simulink model "BrowarModel"  (R2024a)
settings: Solver=ode5  StartTime=0.0  StopTime=inf  FixedStep=0.1  RelTol=1e-3
undefined symbols (not defined in the file or in its folder): localhost, Matrikon, OI
libraries: opclib x24
(part 6 of 9)

== system BrowarModel/Mlyn browarniany/Mlyn browarniany/Zawor doplywu slodu ==
  note: Zawor doplywu slodu
  note: Uszkodzenie:
      | Brak materialu
  note: Uszkodzenie:
      | Dlawienie przeplywu w zaworze
  note: Uszkodzenie:
      | Przeciek wewnetrzny w zaworze
  note: Uszkodzenie:
      | Wyciek zewnetrzny w zaworze
  Sterowanie : Inport
  Dlawienie : Inport  Port=2
  Przeciek : Inport  Port=3
  Wyciek : Inport  Port=4
  Brak : Inport  Port=5
  Const : Constant  Value=100
  Const1 : Constant  Value=100
  Const2 : Constant  Value=100
  GUIMon : Gain
  Gain : Gain  Gain=1/100
  Gain1 : Gain  Gain=1/100
  Gain2 : Gain  Gain=1/100
  Integer Delay : Delay  DelayLength=15
  Napelnianie m3/s : Gain  Gain=Fmax/100
  Product : Product  RndMeth=Zero
  Product1 : Product  RndMeth=Zero
  Product2 : Product  RndMeth=Zero
  Relay : Relay  OnOutputValue=100
  Sat (0-100) : Saturate  UpperLimit=100  LowerLimit=0
  Sat dlawienie (0-100) : Saturate  UpperLimit=100  LowerLimit=0
  Sat przecieku (0-100) : Saturate  UpperLimit=100  LowerLimit=0
  Sat uszk (0-100) : Saturate  UpperLimit=100  LowerLimit=0
  Sat wyciek (0-100) : Saturate  UpperLimit=100  LowerLimit=0
  Sum : Sum  Inputs=|+-
  Sum1 : Sum  Inputs=|++
  Sum2 : Sum  Inputs=|+-
  Sum3 : Sum  Inputs=|+-
  Sum5 : Sum  Inputs=|++
  Transfer Fcn : TransferFcn  Denominator=[1 1]
  Zaklocenia : Subsystem
  Przeplyw : Outport
  wires:
  Product/1 -> Transfer Fcn/1  "m3/s"
  Const/1 -> Sum/1
  Sat dlawienie (0-100)/1 -> Sum/2
  Sum/1 -> Gain/1
  Transfer Fcn/1 -> Integer Delay/1  "m3/s"
  Sterowanie/1 -> Relay/1
  Dlawienie/1 -> Sat dlawienie (0-100)/1  "[0,100]"
  Sat (0-100)/1 -> Napelnianie m3/s/1
  Sum1/1 -> Sat (0-100)/1
  Relay/1 -> GUIMon/1
  Przeciek/1 -> Sat przecieku (0-100)/1
  Sat przecieku (0-100)/1 -> Sum1/2
  Wyciek/1 -> Sat wyciek (0-100)/1
  Const1/1 -> Sum2/1
  Sat wyciek (0-100)/1 -> Sum2/2
  Integer Delay/1 -> Product1/1  "m3/s"
  Product1/1 -> Przeplyw/1
  Sum2/1 -> Gain1/1
  Gain1/1 -> Product1/2
  Product2/1 -> Sum1/1
  GUIMon/1 -> Product2/2
  Brak/1 -> Sat uszk (0-100)/1
  Const2/1 -> Sum3/1
  Sat uszk (0-100)/1 -> Sum3/2
  Sum3/1 -> Gain2/1
  Sum5/1 -> Product/2
  Gain/1 -> Product/1
  Zaklocenia/1(Out) -> Sum5/2
  Gain2/1 -> Product2/1
  Napelnianie m3/s/1 -> Sum5/1, Zaklocenia/1(In)

== system BrowarModel/Mlyn browarniany/ST103/Zaklocenia pomiarowe ==
  Product1 : Product  InputSameDT=on  RndMeth=Zero  SaturateOnIntegerOverflow=on  OutDataTypeStr=Inherit: Same as first input
  Product3 : Product  InputSameDT=on  RndMeth=Zero  SaturateOnIntegerOverflow=on  OutDataTypeStr=Inherit: Same as first input
  Random Number : RandomNumber  Variance=.5  Seed=4365624  SampleTime=0.1
  Transfer Fcn1 : TransferFcn  Denominator=[0.5 1]
  Transfer Fcn2 : TransferFcn  Denominator=[0.5 1]
  Zaklocenia pomiarowe : Constant  Value=ZakloceniaPom
  Out : Outport
  wires:
  Random Number/1 -> Product3/1
  Product3/1 -> Transfer Fcn1/1
  Transfer Fcn1/1 -> Transfer Fcn2/1
  Transfer Fcn2/1 -> Out/1
  Zaklocenia pomiarowe/1 -> Product1/2
  [ZaklPom] -> Product1/1
  Product1/1 -> Product3/2

== system BrowarModel/Mlyn browarniany/ST105/Zaklocenia pomiarowe ==
  Product1 : Product  InputSameDT=on  RndMeth=Zero  SaturateOnIntegerOverflow=on  OutDataTypeStr=Inherit: Same as first input
  Product3 : Product  InputSameDT=on  RndMeth=Zero  SaturateOnIntegerOverflow=on  OutDataTypeStr=Inherit: Same as first input
  Random Number : RandomNumber  Variance=.5  Seed=4365624  SampleTime=0.1
  Transfer Fcn1 : TransferFcn  Denominator=[0.5 1]
  Transfer Fcn2 : TransferFcn  Denominator=[0.5 1]
  Zaklocenia pomiarowe : Constant  Value=ZakloceniaPom
  Out : Outport
  wires:
  Product1/1 -> Product3/2
  [ZaklPom] -> Product1/1
  Zaklocenia pomiarowe/1 -> Product1/2
  Transfer Fcn2/1 -> Out/1
  Transfer Fcn1/1 -> Transfer Fcn2/1
  Product3/1 -> Transfer Fcn1/1
  Random Number/1 -> Product3/1

== system BrowarModel/Mlyn browarniany/TT103/Zaklocenia pomiarowe ==
  Product1 : Product  InputSameDT=on  RndMeth=Zero  SaturateOnIntegerOverflow=on  OutDataTypeStr=Inherit: Same as first input
  Product3 : Product  InputSameDT=on  RndMeth=Zero  SaturateOnIntegerOverflow=on  OutDataTypeStr=Inherit: Same as first input
  Random Number : RandomNumber  Variance=.5  Seed=4365624  SampleTime=0.1
  Transfer Fcn1 : TransferFcn  Denominator=[0.5 1]
  Transfer Fcn2 : TransferFcn  Denominator=[0.5 1]
  Zaklocenia pomiarowe : Constant  Value=ZakloceniaPom
  Out : Outport
  wires:
  Random Number/1 -> Product3/1
  Product3/1 -> Transfer Fcn1/1
  Transfer Fcn1/1 -> Transfer Fcn2/1
  Transfer Fcn2/1 -> Out/1
  Zaklocenia pomiarowe/1 -> Product1/2
  [ZaklPom] -> Product1/1
  Product1/1 -> Product3/2

== system BrowarModel/Mlyn browarniany/TT105/Zaklocenia pomiarowe ==
  Product1 : Product  InputSameDT=on  RndMeth=Zero  SaturateOnIntegerOverflow=on  OutDataTypeStr=Inherit: Same as first input
  Product3 : Product  InputSameDT=on  RndMeth=Zero  SaturateOnIntegerOverflow=on  OutDataTypeStr=Inherit: Same as first input
  Random Number : RandomNumber  Variance=.5  Seed=4365624  SampleTime=0.1
  Transfer Fcn1 : TransferFcn  Denominator=[0.5 1]
  Transfer Fcn2 : TransferFcn  Denominator=[0.5 1]
  Zaklocenia pomiarowe : Constant  Value=ZakloceniaPom
  Out : Outport
  wires:
  Product1/1 -> Product3/2
  [ZaklPom] -> Product1/1
  Zaklocenia pomiarowe/1 -> Product1/2
  Transfer Fcn2/1 -> Out/1
  Transfer Fcn1/1 -> Transfer Fcn2/1
  Product3/1 -> Transfer Fcn1/1
  Random Number/1 -> Product3/1

== system BrowarModel/Schladzacz/TT601/Zaklocenia pomiarowe ==
  Product1 : Product  InputSameDT=on  RndMeth=Zero  SaturateOnIntegerOverflow=on  OutDataTypeStr=Inherit: Same as first input
  Product3 : Product  InputSameDT=on  RndMeth=Zero  SaturateOnIntegerOverflow=on  OutDataTypeStr=Inherit: Same as first input
  Random Number : RandomNumber  Variance=.5  Seed=4365624  SampleTime=0.1
  Transfer Fcn1 : TransferFcn  Denominator=[0.5 1]
  Transfer Fcn2 : TransferFcn  Denominator=[0.5 1]
  Zaklocenia pomiarowe : Constant  Value=ZakloceniaPom
  Out : Outport
  wires:
  Random Number/1 -> Product3/1
  Product3/1 -> Transfer Fcn1/1
  Transfer Fcn1/1 -> Transfer Fcn2/1
  Transfer Fcn2/1 -> Out/1
  Zaklocenia pomiarowe/1 -> Product1/2
  [ZaklPom] -> Product1/1
  Product1/1 -> Product3/2

== system BrowarModel/Schladzacz/TT602/Zaklocenia pomiarowe ==
  Product1 : Product  InputSameDT=on  RndMeth=Zero  SaturateOnIntegerOverflow=on  OutDataTypeStr=Inherit: Same as first input
  Product3 : Product  InputSameDT=on  RndMeth=Zero  SaturateOnIntegerOverflow=on  OutDataTypeStr=Inherit: Same as first input
  Random Number : RandomNumber  Variance=.5  Seed=4365624  SampleTime=0.1
  Transfer Fcn1 : TransferFcn  Denominator=[0.5 1]
  Transfer Fcn2 : TransferFcn  Denominator=[0.5 1]
  Zaklocenia pomiarowe : Constant  Value=ZakloceniaPom
  Out : Outport
  wires:
  Product1/1 -> Product3/2
  [ZaklPom] -> Product1/1
  Zaklocenia pomiarowe/1 -> Product1/2
  Transfer Fcn2/1 -> Out/1
  Transfer Fcn1/1 -> Transfer Fcn2/1
  Product3/1 -> Transfer Fcn1/1
  Random Number/1 -> Product3/1

== system BrowarModel/Schladzacz/TT603/Zaklocenia pomiarowe ==
  Product1 : Product  InputSameDT=on  RndMeth=Zero  SaturateOnIntegerOverflow=on  OutDataTypeStr=Inherit: Same as first input
  Product3 : Product  InputSameDT=on  RndMeth=Zero  SaturateOnIntegerOverflow=on  OutDataTypeStr=Inherit: Same as first input
  Random Number : RandomNumber  Variance=.5  Seed=4365624  SampleTime=0.1
  Transfer Fcn1 : TransferFcn  Denominator=[0.5 1]
  Transfer Fcn2 : TransferFcn  Denominator=[0.5 1]
  Zaklocenia pomiarowe : Constant  Value=ZakloceniaPom
  Out : Outport
  wires:
  Random Number/1 -> Product3/1
  Product3/1 -> Transfer Fcn1/1
  Transfer Fcn1/1 -> Transfer Fcn2/1
  Transfer Fcn2/1 -> Out/1
  Zaklocenia pomiarowe/1 -> Product1/2
  [ZaklPom] -> Product1/1
  Product1/1 -> Product3/2

== system BrowarModel/Schladzacz/TT604/Zaklocenia pomiarowe ==
  Product1 : Product  InputSameDT=on  RndMeth=Zero  SaturateOnIntegerOverflow=on  OutDataTypeStr=Inherit: Same as first input
  Product3 : Product  InputSameDT=on  RndMeth=Zero  SaturateOnIntegerOverflow=on  OutDataTypeStr=Inherit: Same as first input
  Random Number : RandomNumber  Variance=.5  Seed=4365624  SampleTime=0.1
  Transfer Fcn1 : TransferFcn  Denominator=[0.5 1]
  Transfer Fcn2 : TransferFcn  Denominator=[0.5 1]
  Zaklocenia pomiarowe : Constant  Value=ZakloceniaPom
  Out : Outport
  wires:
  Product1/1 -> Product3/2
  [ZaklPom] -> Product1/1
  Zaklocenia pomiarowe/1 -> Product1/2
  Transfer Fcn2/1 -> Out/1
  Transfer Fcn1/1 -> Transfer Fcn2/1
  Product3/1 -> Transfer Fcn1/1
  Random Number/1 -> Product3/1

== system BrowarModel/System dozowania chmielu/PT503/Zaklocenia pomiarowe ==
  Product1 : Product  InputSameDT=on  RndMeth=Zero  SaturateOnIntegerOverflow=on  OutDataTypeStr=Inherit: Same as first input
  Product3 : Product  InputSameDT=on  RndMeth=Zero  SaturateOnIntegerOverflow=on  OutDataTypeStr=Inherit: Same as first input
  Random Number : RandomNumber  Variance=.5  Seed=4365624  SampleTime=0.1
  Transfer Fcn1 : TransferFcn  Denominator=[0.5 1]
  Transfer Fcn2 : TransferFcn  Denominator=[0.5 1]
  Zaklocenia pomiarowe : Constant  Value=ZakloceniaPom
  Out : Outport
  wires:
  Product1/1 -> Product3/2
  [ZaklPom] -> Product1/1
  Zaklocenia pomiarowe/1 -> Product1/2
  Transfer Fcn2/1 -> Out/1
  Transfer Fcn1/1 -> Transfer Fcn2/1
  Product3/1 -> Transfer Fcn1/1
  Random Number/1 -> Product3/1

== system BrowarModel/System dozowania chmielu/System dozowania chmielu/Ruszt dozujacy ==
  note: Ruszt dozujacy
  Pozycja : Inport
  Poziom_w_zbiorniku : Inport  Port=2
  Dot Product : DotProduct  OutDataTypeStr=Inherit: Inherit via internal rule
  Gain : Gain  Gain=20
  Inercja proszku : TransferFcn  Denominator=[0.1 1]
  Parcie proszku na ruszt : Lookup  InputValues=[0, 0.1, 5]  Table=[0, 1, 1]  SaturateOnIntegerOverflow=off
  Pole otwarcia : Lookup  InputValues=[0, 0.015, 0.05, 0.09, 0.1]  Table=[0, 0, 0.0003, 0.001, 0.001]  SaturateOnIntegerOverflow=off
  Saturation : Saturate  UpperLimit=inf  LowerLimit=0
  Przeplyw : Outport
  wires:
  Pozycja/1 -> Pole otwarcia/1  "m"
  Pole otwarcia/1 -> Gain/1
  Poziom_w_zbiorniku/1 -> Parcie proszku na ruszt/1  "m"
  Parcie proszku na ruszt/1 -> Dot Product/2
  Dot Product/1 -> Inercja proszku/1  "m^3/s"
  Inercja proszku/1 -> Saturation/1  "m3/s"
  Saturation/1 -> Przeplyw/1
  Gain/1 -> Dot Product/1

== system BrowarModel/System dozowania chmielu/System dozowania chmielu/Silownik hydrauliczny ==
  note: Silownik hydrauliczny
  Przeplyw zasilanie : Inport
  Uszkodzenie : Inport  Port=2
  Abs1 : Abs  SaturateOnIntegerOverflow=off
  Abs2 : Abs  SaturateOnIntegerOverflow=off
  Add : Sum
  Add1 : Sum
  Add2 : Sum
  Brak przeplywu : Constant  Value=0
  Divide1 : Product  Inputs=*/
  Divide2 : Product  Inputs=/*
  Dot Product : DotProduct  OutDataTypeStr=Inherit: Inherit via internal rule
  Dot Product1 : DotProduct  OutDataTypeStr=Inherit: Inherit via internal rule
  Gain : Gain  Gain=0.1/100
  Inercja : TransferFcn  Denominator=[0.2 1]
  Integrator : Integrator  LimitOutput=on  UpperSaturationLimit=0.1  LowerSaturationLimit=0  ShowSaturationPort=on
  Napelnianie : Saturate  UpperLimit=inf  LowerLimit=0
  Napelnianie1 : Saturate  UpperLimit=inf  LowerLimit=0
  Oproznianie : Saturate  UpperLimit=0  LowerLimit=-inf
  Oproznianie1 : Saturate  UpperLimit=0  LowerLimit=-inf
  Pole tloczyska gdy silownik otwierany : Constant  Value=0.002
  Pole tloczyska gdy silownik zamykany : Constant  Value=0.001
  Sat : Saturate  UpperLimit=100  LowerLimit=0
  Sat1 : Saturate  UpperLimit=0.1  LowerLimit=0
  Switch : Switch  Threshold=0.5  SaturateOnIntegerOverflow=off  InputSameDT=off
  Pozycja : Outport
  Przeplyw pobor : Outport  Port=2
  wires:
  Przeplyw zasilanie/1 -> Napelnianie/1, Oproznianie/1  "m3/s"
  Add/1 -> Inercja/1  "m/s"
  Napelnianie/1 -> Divide2/2
  Divide2/1 -> Add/1  "m/s"
  Divide1/1 -> Add/2  "m/s"
  Oproznianie/1 -> Divide1/1
  Pole tloczyska gdy silownik zamykany/1 -> Divide1/2, Dot Product1/2
  Pole tloczyska gdy silownik otwierany/1 -> Divide2/1, Dot Product/1
  Switch/1 -> Przeplyw pobor/1
  Integrator/2 -> Abs2/1
  Inercja/1 -> Integrator/1, Napelnianie1/1, Oproznianie1/1
  Oproznianie1/1 -> Abs1/1
  Abs1/1 -> Dot Product1/1
  Napelnianie1/1 -> Dot Product/2
  Dot Product/1 -> Add1/1
  Abs2/1 -> Switch/2
  Brak przeplywu/1 -> Switch/1
  Add1/1 -> Switch/3
  Dot Product1/1 -> Add1/2
  Uszkodzenie/1 -> Sat/1
  Integrator/1 -> Add2/2  "m"
  Add2/1 -> Sat1/1
  Sat/1 -> Gain/1
  Sat1/1 -> Pozycja/1
  Gain/1 -> Add2/1

== system BrowarModel/System dozowania chmielu/System dozowania chmielu/Sterownik rusztu ==
  note: Sterownik rusztu
  Pozycja rusztu : Inport
  Nastawa : Inport  Port=2
  Char rusztu (reset) : Lookup  InputValues=|  Table=|  SaturateOnIntegerOverflow=off
      InputValues=|
      | [1
      | 2
      | 3
      | 4
      | 5
      | 6
      | 7
      | 8
      | 9
      | 10
      | 11
      | 12
      | 13
      | 14
      | 15
      | 16
      | 17
      | 18
      | 19
      | 20
      | 21
      | 22
      | 23
      | 24
      | 25
      | 26
      | 27
      | 28
      | 29
      | 30
      | 31
      | 32
      | 33
      | 34
      | 35
      | 36
      | 37
      | 38
      | 39
      | 40
      | 41
      | 42
      | 43
      | 44
      | 45
      | 46
      | 47
      | 48
      | 49
      | 50
      | 51
      | 52
      | 53
      | 54
      | 55
      | 56
      | 57
      | 58
      | 59
      | 60
      | 61
      | 62
      | 63
      | 64
      | 65
      | 66
      | 67
      | 68
      | 69
      | 70
      | 71
      | 72
      | 73
      | 74
      | 75
      | 76
      | 77
      | 78
      | 79
      | 80
      | 81
      | 82
      | 83
      | 84
      | 85
      | 86
      | 87
      | 88
      | 89
      | 90
      | 91
      | 92
      | 93
      | 94
      | 95
      | 96
      | 97
      | 98
      | 99
      | 100]
      Table=|
      | [9.24
      | 9.55
      | 9.84
      | 10.13
      | 10.44
      | 10.76
      | 11.11
      | 11.47
      | 11.84
      | 12.24
      | 12.65
      | 13.08
      | 13.52
      | 13.98
      | 14.45
      | 14.94
      | 15.44
      | 15.95
      | 16.48
      | 17.02
      | 17.58
      | 18.15
      | 18.72
      | 19.32
      | 19.92
      | 20.53
      | 21.16
      | 21.80
      | 22.44
      | 23.10
      | 23.77
      | 24.45
      | 25.14
      | 25.84
      | 26.56
      | 27.28
      | 28.01
      | 28.75
      | 29.50
      | 30.26
      | 31.03
      | 31.80
      | 32.59
      | 33.39
      | 34.19
      | 35.00
      | 35.83
      | 36.66
      | 37.50
      | 38.35
      | 39.20
      | 40.07
      | 40.94
      | 41.82
      | 42.71
      | 43.61
      | 44.51
      | 45.42
      | 46.35
      | 47.27
      | 48.21
      | 49.15
      | 50.10
      | 51.06
      | 52.03
      | 53.00
      | 53.98
      | 54.97
      | 55.97
      | 56.97
      | 57.98
      | 59.00
      | 60.02
      | 61.05
      | 62.09
      | 63.13
      | 64.18
      | 65.24
      | 66.31
      | 67.38
      | 68.46
      | 69.54
      | 70.63
      | 71.73
      | 72.84
      | 73.95
      | 75.06
      | 76.19
      | 77.32
      | 78.46
      | 79.60
      | 80.75
      | 81.90
      | 83.06
      | 84.23
      | 85.40
      | 86.58
      | 87.77
      | 88.96
      | 90.16]
  Char rusztu (set) : Lookup  InputValues=|  Table=|  SaturateOnIntegerOverflow=off
      InputValues=|
      | [1
      | 2
      | 3
      | 4
      | 5
      | 6
      | 7
      | 8
      | 9
      | 10
      | 11
      | 12
      | 13
      | 14
      | 15
      | 16
      | 17
      | 18
      | 19
      | 20
      | 21
      | 22
      | 23
      | 24
      | 25
      | 26
      | 27
      | 28
      | 29
      | 30
      | 31
      | 32
      | 33
      | 34
      | 35
      | 36
      | 37
      | 38
      | 39
      | 40
      | 41
      | 42
      | 43
      | 44
      | 45
      | 46
      | 47
      | 48
      | 49
      | 50
      | 51
      | 52
      | 53
      | 54
      | 55
      | 56
      | 57
      | 58
      | 59
      | 60
      | 61
      | 62
      | 63
      | 64
      | 65
      | 66
      | 67
      | 68
      | 69
      | 70
      | 71
      | 72
      | 73
      | 74
      | 75
      | 76
      | 77
      | 78
      | 79
      | 80
      | 81
      | 82
      | 83
      | 84
      | 85
      | 86
      | 87
      | 88
      | 89
      | 90
      | 91
      | 92
      | 93
      | 94
      | 95
      | 96
      | 97
      | 98
      | 99
      | 100]
      Table=|
      | [7.50
      | 7.66
      | 7.80
      | 7.95
      | 8.10
      | 8.26
      | 8.43
      | 8.61
      | 8.80
      | 9.00
      | 9.20
      | 9.42
      | 9.64
      | 9.87
      | 10.11
      | 10.35
      | 10.60
      | 10.86
      | 11.12
      | 11.39
      | 11.67
      | 11.95
      | 12.24
      | 12.54
      | 12.84
      | 13.15
      | 13.46
      | 13.78
      | 14.10
      | 14.43
      | 14.77
      | 15.11
      | 15.45
      | 15.80
      | 16.16
      | 16.52
      | 16.88
      | 17.25
      | 17.63
      | 18.01
      | 18.39
      | 18.78
      | 19.17
      | 19.57
      | 19.98
      | 20.38
      | 20.79
      | 21.21
      | 21.63
      | 22.05
      | 22.48
      | 22.91
      | 23.35
      | 23.79
      | 24.23
      | 24.68
      | 25.14
      | 25.59
      | 26.05
      | 26.52
      | 26.98
      | 27.46
      | 27.93
      | 28.41
      | 28.89
      | 29.38
      | 29.87
      | 30.37
      | 30.86
      | 31.37
      | 31.87
      | 32.38
      | 32.89
      | 33.41
      | 33.92
      | 34.45
      | 34.97
      | 35.50
      | 36.03
      | 36.57
      | 37.11
      | 37.65
      | 38.20
      | 38.75
      | 39.30
      | 39.85
      | 40.41
      | 40.97
      | 41.54
      | 42.11
      | 42.68
      | 43.25
      | 43.83
      | 44.41
      | 45.00
      | 45.58
      | 46.17
      | 46.77
      | 47.36
      | 47.96]
  Constant : Constant  Value=0
  Gain : Gain  Gain=0.001
  Gain1 : Gain  Gain=0.001
  Logical Operator : Logic  Operator=OR  AllPortsSameDT=off
  Logical Operator1 : Logic  AllPortsSameDT=off
  Logical Operator2 : Logic  Operator=NOT  AllPortsSameDT=off
  Logical Operator3 : Logic  AllPortsSameDT=off
  Memory : Memory
  Relational Operator : RelationalOperator  Operator=<=  InputSameDT=off
  Relational Operator1 : RelationalOperator  InputSameDT=off
  Relational Operator2 : RelationalOperator  Operator=>  InputSameDT=off
  Rounding Function : Rounding
  Sterowanie zaworem : Outport
  wires:
  Nastawa/1 -> Rounding Function/1
  Char rusztu (set)/1 -> Gain/1  "%"
  Char rusztu (reset)/1 -> Gain1/1  "%"
  Relational Operator/1 -> Logical Operator/1
  Logical Operator/1 -> Memory/1, Logical Operator3/1
  Memory/1 -> Logical Operator1/1
  Logical Operator1/1 -> Logical Operator/2
  Relational Operator1/1 -> Logical Operator2/1
  Logical Operator2/1 -> Logical Operator1/2
  Pozycja rusztu/1 -> Relational Operator/1, Relational Operator1/1  "m"
  Logical Operator3/1 -> Sterowanie zaworem/1
  Relational Operator2/1 -> Logical Operator3/2
  Constant/1 -> Relational Operator2/2
  Gain/1 -> Relational Operator/2  "m"
  Gain1/1 -> Relational Operator1/2  "m"
  Rounding Function/1 -> Char rusztu (set)/1, Char rusztu (reset)/1, Relational Operator2/1

== system BrowarModel/System dozowania chmielu/System dozowania chmielu/Waga ==
  note: Waga
  note: Uszkodzenie mechanizmu
      | oprozniania wago
  Doplyw : Inport
  Oproznianie : Inport  Port=2
  Uszkodzenie oprozniania : Inport  Port=3
  1/Gestosc : Gain  Gain=1/1000
  Dot Product : DotProduct  OutDataTypeStr=Inherit: Inherit via internal rule
  Dynamika oprozniania : Gain  Gain=0.75
  Gestosc : Gain  Gain=1000
  Integrator : Integrator  LimitOutput=on  UpperSaturationLimit=100  LowerSaturationLimit=0
  Logical Operator : Logic  Operator=NOT  AllPortsSameDT=off
  Poz_dol : RelationalOperator  InputSameDT=off
  Poz_gora : RelationalOperator  Operator=<=  InputSameDT=off
  Pozycja dol : Constant  Value=0.9
  Pozycja gora : Constant  Value=0.1
  Product : Product  RndMeth=Zero
  Relay : Relay
  Relay1 : Relay
  Saturation : Saturate  UpperLimit=inf  LowerLimit=0
  Saturation1 : Saturate  UpperLimit=100  LowerLimit=0
  Sum : Sum  Inputs=|+-
  Sum1 : Sum
  Transfer Fcn : TransferFcn  Denominator=[1 1]
  Transport Delay : TransportDelay  DelayTime=1.5
  Wspolczynnik dynamiczny : Gain  Gain=.2
  Masa : Outport
  Odplyw chmielu : Outport  Port=2
  Poz dol : Outport  Port=3
  Poz gora : Outport  Port=4
  wires:
  Gestosc/1 -> Transport Delay/1  "kg/s"
  Transport Delay/1 -> Wspolczynnik dynamiczny/1, Sum/1
  Saturation/1 -> Gestosc/1  "m^3/s"
  Integrator/1 -> Dynamika oprozniania/1, Sum1/2
  Wspolczynnik dynamiczny/1 -> Sum1/1
  Doplyw/1 -> Saturation/1
  Sum1/1 -> Saturation1/1  "kg"
  Sum/1 -> Integrator/1
  Dot Product/1 -> Sum/2, 1/Gestosc/1
  Dynamika oprozniania/1 -> Dot Product/2
  1/Gestosc/1 -> Odplyw chmielu/1
  Saturation1/1 -> Masa/1  "kg"
  Poz_dol/1 -> Poz dol/1, Dot Product/1
  Poz_gora/1 -> Poz gora/1
  Pozycja dol/1 -> Poz_dol/2
  Pozycja gora/1 -> Poz_gora/2
  Transfer Fcn/1 -> Poz_dol/1, Poz_gora/1
  Oproznianie/1 -> Relay/1
  Uszkodzenie oprozniania/1 -> Relay1/1
  Relay1/1 -> Logical Operator/1
  Product/1 -> Transfer Fcn/1
  Relay/1 -> Product/1
  Logical Operator/1 -> Product/2

== system BrowarModel/System dozowania chmielu/System dozowania chmielu/Zasilacz hydrauliczny ==
  note: obr/min
  note: Zasilacz hydrauliczny
  note: Uszkodzenie:
      | Spadek cisnienia zasilania
  note: Uszkodzenie silnika pompy
  Zalaczenie pompy : Inport
  Przeplyw_pobor : Inport  Port=2
  Spadek cisnienia : Inport  Port=3
  Uszkodzenie silnika : Inport  Port=4
  Charakterystyka pompy F=f(P) (max 0.0001 m^3/s) : Lookup  InputValues=[0, 300]  Table=[0,0.0001]  SaturateOnIntegerOverflow=off
  Charakterystyka pompy P=f(obr) (max 300 kPa) : Lookup  InputValues=[0, 1440]  Table=[0,300]  SaturateOnIntegerOverflow=off
  Const1 : Constant  Value=100
  GUIMon : Gain
  Gain : Gain  Gain=1/100
  Gain1 : Gain  Gain=1/100
  Inercja wirnika : TransferFcn  Denominator=[0.5 1]
  Math Function : Math  Operator=square  SignedPower=on
  Obroty nominalne pompy : Gain  Gain=1440
  Opor : Gain  Gain=250 / ((0.0001)^2)
  Product1 : Product  RndMeth=Zero
  Relay : Relay  OnOutputValue=100
  Relay1 : Relay  OnOutputValue=0  OffOutputValue=1
  Sat uszk : Saturate  UpperLimit=100  LowerLimit=0
  Saturation : Saturate  UpperLimit=inf  LowerLimit=0
  Spadek obrotow pompy (od obciazenia) : Lookup  InputValues=[0, 300]  Table=[0,100]  SaturateOnIntegerOverflow=off
  Sum1 : Sum  Inputs=|+-
  Sum2 : Sum  Inputs=|+-
  Sum3 : Sum  Inputs=|+-
  Wplyw uszkodzenia : DotProduct  OutDataTypeStr=Inherit: Inherit via internal rule
  Max przeplyw zasilanie : Outport
  Cisnienie zasilania : Outport  Port=2
  wires:
  Obroty nominalne pompy/1 -> Sum2/1
  Sum2/1 -> Inercja wirnika/1
  Spadek obrotow pompy (od obciazenia)/1 -> Sum2/2  "obr/min"
  Inercja wirnika/1 -> Charakterystyka pompy P=f(obr) (max 300 kPa)/1  "obr/min"
  Charakterystyka pompy F=f(P) (max 0.0001 m^3/s)/1 -> Max przeplyw zasilanie/1  "m^3/s"
  Sum1/1 -> Saturation/1
  Opor/1 -> Sum1/2  "kPa"
  Saturation/1 -> Spadek obrotow pompy (od obciazenia)/1, Cisnienie zasilania/1, Charakterystyka pompy F=f(P) (max 0.0001 m^3/s)/1  "kPa"
  Math Function/1 -> Opor/1
  Zalaczenie pompy/1 -> Relay/1
  Przeplyw_pobor/1 -> Math Function/1
  Spadek cisnienia/1 -> Sat uszk/1
  Charakterystyka pompy P=f(obr) (max 300 kPa)/1 -> Product1/2  "kPa"
  Product1/1 -> Sum1/1  "kPa"
  Sat uszk/1 -> Sum3/2
  Const1/1 -> Sum3/1
  Sum3/1 -> Gain/1
  Wplyw uszkodzenia/1 -> Obroty nominalne pompy/1
  Relay/1 -> GUIMon/1
  Uszkodzenie silnika/1 -> Relay1/1
  Relay1/1 -> Wplyw uszkodzenia/2
  Gain/1 -> Product1/1
  GUIMon/1 -> Gain1/1
  Gain1/1 -> Wplyw uszkodzenia/1

== system BrowarModel/System dozowania chmielu/System dozowania chmielu/Zasobnik ==
  note: Zasobnik dozownika chmielu
  note: Uszkodzenie:
      | Wyciek z zasobnika dozownika
  Doplyw : Inport
  Odplyw : Inport  Port=2
  Wyciek : Inport  Port=3
  Char. zbiornika : Lookup  InputValues="[0.000\t0.003\t0.010\t0.023\t0.046\t0.079\t0.125\t0.186\t0.264\t0.362\t0.480\t0.622\t0.790\t0.972\t1.172\t1.372\t1.572\t1.772\t1.972\t2.172\t2.372\t2.572\t2.772\t2.972\t3.172\t3.372\t3.572\t3.772\t3.972\t4.172\t4.372\t4.572\t4.772\t4.972]"  Table="[0\t0.1\t0.2\t0.3\t0.4\t0.5\t0.6\t0.7\t0.8\t0.9\t1\t1.1\t1.2\t1.3\t1.4\t1.5\t1.6\t1.7\t1.8\t1.9\t2\t2.1\t2.2\t2.3\t2.4\t2.5\t2.6\t2.7\t2.8\t2.9\t3\t3.1\t3.2\t3.3]"  SaturateOnIntegerOverflow=off
  Detektory poziomu : Subsystem
  Integrator (max = 4.92m3) : Integrator  LimitOutput=on  UpperSaturationLimit=4.92  LowerSaturationLimit=0
  Max wyciek : Gain  Gain=0.01
  Product : Product  RndMeth=Zero
  Sat doplyw (F>=0) : Saturate  UpperLimit=inf  LowerLimit=0
  Sat odplyw (F>=0) : Saturate  UpperLimit=inf  LowerLimit=0
  Sat wyciek (0-1) : Saturate  UpperLimit=1  LowerLimit=0
  Sum : Sum  Inputs=|+-
  Sum1 : Sum  Inputs=|+-
  Wyciek char : Lookup  InputValues=[0, 0.5, 0.6, 1]  Table=[0, 0, 1, 1]  SaturateOnIntegerOverflow=off
  Poziom : Outport
  Poziom HI : Outport  Port=2
  Poziom LO : Outport  Port=3
  wires:
  Doplyw/1 -> Sat doplyw (F>=0)/1  "m3/s"
  Odplyw/1 -> Sat odplyw (F>=0)/1  "m3/s"
  Integrator (max = 4.92m3)/1 -> Char. zbiornika/1  "m3"
  Char. zbiornika/1 -> Poziom/1, Detektory poziomu/1(Poziom), Wyciek char/1  "m"
  Sat doplyw (F>=0)/1 -> Sum/1
  Sat odplyw (F>=0)/1 -> Sum/2
  Sum1/1 -> Integrator (max = 4.92m3)/1
  Sum/1 -> Sum1/1  "m3/s"
  Wyciek/1 -> Sat wyciek (0-1)/1  "[0,1]"
  Product/1 -> Sum1/2  "m3/h"
  Detektory poziomu/2(Poziom niski) -> Poziom LO/1
  Detektory poziomu/1(Poziom  wysoki) -> Poziom HI/1
  Sat wyciek (0-1)/1 -> Product/1
  Wyciek char/1 -> Max wyciek/1  "[0..1]"
  Max wyciek/1 -> Product/2  "m3/h"

== system BrowarModel/System dozowania chmielu/System dozowania chmielu/Zawor doplywu chmielu ==
  note: Zawor doplywu slodu
  note: Uszkodzenie:
      | Brak materialu
  note: Uszkodzenie:
      | Dlawienie przeplywu w zaworze
  note: Uszkodzenie:
      | Przeciek wewnetrzny w zaworze
  note: Uszkodzenie:
      | Wyciek zewnetrzny w zaworze
  Sterowanie : Inport
  Dlawienie : Inport  Port=2
  Przeciek : Inport  Port=3
  Wyciek : Inport  Port=4
  Brak : Inport  Port=5
  Const : Constant  Value=100
  Const1 : Constant  Value=100
  Const2 : Constant  Value=100
  GUIMon : Gain
  Gain : Gain  Gain=1/100
  Gain1 : Gain  Gain=1/100
  Gain2 : Gain  Gain=1/100
  Integer Delay : Delay  DelayLength=15
  Napelnianie m3/s : Gain  Gain=Fmax/100
  Product : Product  RndMeth=Zero
  Product1 : Product  RndMeth=Zero
  Product2 : Product  RndMeth=Zero
  Relay : Relay  OnOutputValue=100
  Sat (0-100) : Saturate  UpperLimit=100  LowerLimit=0
  Sat dlawienie (0-100) : Saturate  UpperLimit=100  LowerLimit=0
  Sat przecieku (0-100) : Saturate  UpperLimit=100  LowerLimit=0
  Sat uszk (0-100) : Saturate  UpperLimit=100  LowerLimit=0
  Sat wyciek (0-100) : Saturate  UpperLimit=100  LowerLimit=0
  Sum : Sum  Inputs=|+-
  Sum1 : Sum  Inputs=|++
  Sum2 : Sum  Inputs=|+-
  Sum3 : Sum  Inputs=|+-
  Sum5 : Sum  Inputs=|++
  Transfer Fcn : TransferFcn  Denominator=[1 1]
  Zaklocenia : Subsystem
  Przeplyw : Outport
  wires:
  Product/1 -> Transfer Fcn/1  "m3/s"
  Const/1 -> Sum/1
  Sat dlawienie (0-100)/1 -> Sum/2
  Sum/1 -> Gain/1
  Transfer Fcn/1 -> Integer Delay/1  "m3/s"
  Sterowanie/1 -> Relay/1
  Dlawienie/1 -> Sat dlawienie (0-100)/1  "[0,100]"
  Sat (0-100)/1 -> Napelnianie m3/s/1
  Sum1/1 -> Sat (0-100)/1
  Relay/1 -> GUIMon/1
  Przeciek/1 -> Sat przecieku (0-100)/1
  Sat przecieku (0-100)/1 -> Sum1/2
  Wyciek/1 -> Sat wyciek (0-100)/1
  Const1/1 -> Sum2/1
  Sat wyciek (0-100)/1 -> Sum2/2
  Integer Delay/1 -> Product1/1  "m3/s"
  Product1/1 -> Przeplyw/1
  Sum2/1 -> Gain1/1
  Gain1/1 -> Product1/2
  Product2/1 -> Sum1/1
  GUIMon/1 -> Product2/2
  Brak/1 -> Sat uszk (0-100)/1
  Const2/1 -> Sum3/1
  Sat uszk (0-100)/1 -> Sum3/2
  Sum3/1 -> Gain2/1
  Napelnianie m3/s/1 -> Sum5/1, Zaklocenia/1(In)
  Sum5/1 -> Product/2
  Gain/1 -> Product/1
  Zaklocenia/1(Out) -> Sum5/2
  Gain2/1 -> Product2/1

== system BrowarModel/System dozowania chmielu/System dozowania chmielu/Zawor trojdrozny ==
  note: Zawor trojdrozny
  Sterowanie rusztem : Inport
  Przeplyw zasilanie : Inport  Port=2
  Dot Product : DotProduct  OutDataTypeStr=Inherit: Inherit via internal rule
  Relay : Relay  OffOutputValue=-1
  Transfer Fcn : TransferFcn  Denominator=[0.1 1]
  Przeplyw sterowanie : Outport
  wires:
  Sterowanie rusztem/1 -> Relay/1
  Relay/1 -> Dot Product/2
  Przeplyw zasilanie/1 -> Dot Product/1
  Dot Product/1 -> Transfer Fcn/1
  Transfer Fcn/1 -> Przeplyw sterowanie/1

== system BrowarModel/System dozowania chmielu/WT505/Zaklocenia pomiarowe ==
  Product1 : Product  InputSameDT=on  RndMeth=Zero  SaturateOnIntegerOverflow=on  OutDataTypeStr=Inherit: Same as first input
  Product3 : Product  InputSameDT=on  RndMeth=Zero  SaturateOnIntegerOverflow=on  OutDataTypeStr=Inherit: Same as first input
  Random Number : RandomNumber  Variance=.04  Seed=4365624  SampleTime=0.1
  Transfer Fcn1 : TransferFcn  Denominator=[0.5 1]
  Transfer Fcn2 : TransferFcn  Denominator=[0.5 1]
  Zaklocenia pomiarowe : Constant  Value=ZakloceniaPom
  Out : Outport
  wires:
  Random Number/1 -> Product3/1
  Product3/1 -> Transfer Fcn1/1
  Transfer Fcn1/1 -> Transfer Fcn2/1
  Transfer Fcn2/1 -> Out/1
  Zaklocenia pomiarowe/1 -> Product1/2
  [ZaklPom] -> Product1/1
  Product1/1 -> Product3/2

== system BrowarModel/System dozowania chmielu/XT504/Zaklocenia pomiarowe ==
  Product1 : Product  InputSameDT=on  RndMeth=Zero  SaturateOnIntegerOverflow=on  OutDataTypeStr=Inherit: Same as first input
  Product3 : Product  InputSameDT=on  RndMeth=Zero  SaturateOnIntegerOverflow=on  OutDataTypeStr=Inherit: Same as first input
  Random Number : RandomNumber  Variance=.5  Seed=4365624  SampleTime=0.1
  Transfer Fcn1 : TransferFcn  Denominator=[0.5 1]
  Transfer Fcn2 : TransferFcn  Denominator=[0.5 1]
  Zaklocenia pomiarowe : Constant  Value=ZakloceniaPom
  Out : Outport
  wires:
  Random Number/1 -> Product3/1
  Product3/1 -> Transfer Fcn1/1
  Transfer Fcn1/1 -> Transfer Fcn2/1
  Transfer Fcn2/1 -> Out/1
  Zaklocenia pomiarowe/1 -> Product1/2
  [ZaklPom] -> Product1/1
  Product1/1 -> Product3/2

== system BrowarModel/System dozowania drozdzy/PT803/Zaklocenia pomiarowe ==
  Product1 : Product  InputSameDT=on  RndMeth=Zero  SaturateOnIntegerOverflow=on  OutDataTypeStr=Inherit: Same as first input
  Product3 : Product  InputSameDT=on  RndMeth=Zero  SaturateOnIntegerOverflow=on  OutDataTypeStr=Inherit: Same as first input
  Random Number : RandomNumber  Variance=.5  Seed=4365624  SampleTime=0.1
  Transfer Fcn1 : TransferFcn  Denominator=[0.5 1]
  Transfer Fcn2 : TransferFcn  Denominator=[0.5 1]
  Zaklocenia pomiarowe : Constant  Value=ZakloceniaPom
  Out : Outport
  wires:
  Product1/1 -> Product3/2
  [ZaklPom] -> Product1/1
  Zaklocenia pomiarowe/1 -> Product1/2
  Transfer Fcn2/1 -> Out/1
  Transfer Fcn1/1 -> Transfer Fcn2/1
  Product3/1 -> Transfer Fcn1/1
  Random Number/1 -> Product3/1

== system BrowarModel/System dozowania drozdzy/System dozowania drozdzy/Ruszt dozujacy ==
  note: Ruszt dozujacy
  Pozycja : Inport
  Poziom_w_zbiorniku : Inport  Port=2
  Dot Product : DotProduct  OutDataTypeStr=Inherit: Inherit via internal rule
  Gain : Gain  Gain=20
  Inercja proszku : TransferFcn  Denominator=[0.1 1]
  Parcie proszku na ruszt : Lookup  InputValues=[0, 0.1, 5]  Table=[0, 1, 1]  SaturateOnIntegerOverflow=off
  Pole otwarcia : Lookup  InputValues=[0, 0.015, 0.05, 0.09, 0.1]  Table=[0, 0, 0.0003, 0.001, 0.001]  SaturateOnIntegerOverflow=off
  Saturation : Saturate  UpperLimit=inf  LowerLimit=0
  Przeplyw : Outport
  wires:
  Gain/1 -> Dot Product/1
  Saturation/1 -> Przeplyw/1
  Inercja proszku/1 -> Saturation/1  "m3/s"
  Dot Product/1 -> Inercja proszku/1  "m^3/s"
  Parcie proszku na ruszt/1 -> Dot Product/2
  Poziom_w_zbiorniku/1 -> Parcie proszku na ruszt/1  "m"
  Pole otwarcia/1 -> Gain/1
  Pozycja/1 -> Pole otwarcia/1  "m"

== system BrowarModel/System dozowania drozdzy/System dozowania drozdzy/Silownik hydrauliczny ==
  note: Silownik hydrauliczny
  Przeplyw zasilanie : Inport
  Uszkodzenie : Inport  Port=2
  Abs1 : Abs  SaturateOnIntegerOverflow=off
  Abs2 : Abs  SaturateOnIntegerOverflow=off
  Add : Sum
  Add1 : Sum
  Add2 : Sum
  Brak przeplywu : Constant  Value=0
  Divide1 : Product  Inputs=*/
  Divide2 : Product  Inputs=/*
  Dot Product : DotProduct  OutDataTypeStr=Inherit: Inherit via internal rule
  Dot Product1 : DotProduct  OutDataTypeStr=Inherit: Inherit via internal rule
  Gain : Gain  Gain=0.1/100
  Inercja : TransferFcn  Denominator=[0.2 1]
  Integrator : Integrator  LimitOutput=on  UpperSaturationLimit=0.1  LowerSaturationLimit=0  ShowSaturationPort=on
  Napelnianie : Saturate  UpperLimit=inf  LowerLimit=0
  Napelnianie1 : Saturate  UpperLimit=inf  LowerLimit=0
  Oproznianie : Saturate  UpperLimit=0  LowerLimit=-inf
  Oproznianie1 : Saturate  UpperLimit=0  LowerLimit=-inf
  Pole tloczyska gdy silownik otwierany : Constant  Value=0.002
  Pole tloczyska gdy silownik zamykany : Constant  Value=0.001
  Sat : Saturate  UpperLimit=100  LowerLimit=0
  Sat1 : Saturate  UpperLimit=0.1  LowerLimit=0
  Switch : Switch  Threshold=0.5  SaturateOnIntegerOverflow=off  InputSameDT=off
  Pozycja : Outport
  Przeplyw pobor : Outport  Port=2
  wires:
  Przeplyw zasilanie/1 -> Napelnianie/1, Oproznianie/1  "m3/s"
  Add/1 -> Inercja/1  "m/s"
  Napelnianie/1 -> Divide2/2
  Divide2/1 -> Add/1  "m/s"
  Divide1/1 -> Add/2  "m/s"
  Oproznianie/1 -> Divide1/1
  Pole tloczyska gdy silownik zamykany/1 -> Divide1/2, Dot Product1/2
  Pole tloczyska gdy silownik otwierany/1 -> Divide2/1, Dot Product/1
  Switch/1 -> Przeplyw pobor/1
  Integrator/2 -> Abs2/1
  Inercja/1 -> Integrator/1, Napelnianie1/1, Oproznianie1/1
  Oproznianie1/1 -> Abs1/1
  Abs1/1 -> Dot Product1/1
  Napelnianie1/1 -> Dot Product/2
  Dot Product/1 -> Add1/1
  Abs2/1 -> Switch/2
  Brak przeplywu/1 -> Switch/1
  Add1/1 -> Switch/3
  Dot Product1/1 -> Add1/2
  Uszkodzenie/1 -> Sat/1
  Integrator/1 -> Add2/2  "m"
  Add2/1 -> Sat1/1
  Sat/1 -> Gain/1
  Sat1/1 -> Pozycja/1
  Gain/1 -> Add2/1

== system BrowarModel/System dozowania drozdzy/System dozowania drozdzy/Sterownik rusztu ==
  note: Sterownik rusztu
  Pozycja rusztu : Inport
  Nastawa : Inport  Port=2
  Char rusztu (reset) : Lookup  InputValues=|  Table=|  SaturateOnIntegerOverflow=off
      InputValues=|
      | [1
      | 2
      | 3
      | 4
      | 5
      | 6
      | 7
      | 8
      | 9
      | 10
      | 11
      | 12
      | 13
      | 14
      | 15
      | 16
      | 17
      | 18
      | 19
      | 20
      | 21
      | 22
      | 23
      | 24
      | 25
      | 26
      | 27
      | 28
      | 29
      | 30
      | 31
      | 32
      | 33
      | 34
      | 35
      | 36
      | 37
      | 38
      | 39
      | 40
      | 41
      | 42
      | 43
      | 44
      | 45
      | 46
      | 47
      | 48
      | 49
      | 50
      | 51
      | 52
      | 53
      | 54
      | 55
      | 56
      | 57
      | 58
      | 59
      | 60
      | 61
      | 62
      | 63
      | 64
      | 65
      | 66
      | 67
      | 68
      | 69
      | 70
      | 71
      | 72
      | 73
      | 74
      | 75
      | 76
      | 77
      | 78
      | 79
      | 80
      | 81
      | 82
      | 83
      | 84
      | 85
      | 86
      | 87
      | 88
      | 89
      | 90
      | 91
      | 92
      | 93
      | 94
      | 95
      | 96
      | 97
      | 98
      | 99
      | 100]
      Table=|
      | [9.24
      | 9.55
      | 9.84
      | 10.13
      | 10.44
      | 10.76
      | 11.11
      | 11.47
      | 11.84
      | 12.24
      | 12.65
      | 13.08
      | 13.52
      | 13.98
      | 14.45
      | 14.94
      | 15.44
      | 15.95
      | 16.48
      | 17.02
      | 17.58
      | 18.15
      | 18.72
      | 19.32
      | 19.92
      | 20.53
      | 21.16
      | 21.80
      | 22.44
      | 23.10
      | 23.77
      | 24.45
      | 25.14
      | 25.84
      | 26.56
      | 27.28
      | 28.01
      | 28.75
      | 29.50
      | 30.26
      | 31.03
      | 31.80
      | 32.59
      | 33.39
      | 34.19
      | 35.00
      | 35.83
      | 36.66
      | 37.50
      | 38.35
      | 39.20
      | 40.07
      | 40.94
      | 41.82
      | 42.71
      | 43.61
      | 44.51
      | 45.42
      | 46.35
      | 47.27
      | 48.21
      | 49.15
      | 50.10
      | 51.06
      | 52.03
      | 53.00
      | 53.98
      | 54.97
      | 55.97
      | 56.97
      | 57.98
      | 59.00
      | 60.02
      | 61.05
      | 62.09
      | 63.13
      | 64.18
      | 65.24
      | 66.31
      | 67.38
      | 68.46
      | 69.54
      | 70.63
      | 71.73
      | 72.84
      | 73.95
      | 75.06
      | 76.19
      | 77.32
      | 78.46
      | 79.60
      | 80.75
      | 81.90
      | 83.06
      | 84.23
      | 85.40
      | 86.58
      | 87.77
      | 88.96
      | 90.16]
  Char rusztu (set) : Lookup  InputValues=|  Table=|  SaturateOnIntegerOverflow=off
      InputValues=|
      | [1
      | 2
      | 3
      | 4
      | 5
      | 6
      | 7
      | 8
      | 9
      | 10
      | 11
      | 12
      | 13
      | 14
      | 15
      | 16
      | 17
      | 18
      | 19
      | 20
      | 21
      | 22
      | 23
      | 24
      | 25
      | 26
      | 27
      | 28
      | 29
      | 30
      | 31
      | 32
      | 33
      | 34
      | 35
      | 36
      | 37
      | 38
      | 39
      | 40
      | 41
      | 42
      | 43
      | 44
      | 45
      | 46
      | 47
      | 48
      | 49
      | 50
      | 51
      | 52
      | 53
      | 54
      | 55
      | 56
      | 57
      | 58
      | 59
      | 60
      | 61
      | 62
      | 63
      | 64
      | 65
      | 66
      | 67
      | 68
      | 69
      | 70
      | 71
      | 72
      | 73
      | 74
      | 75
      | 76
      | 77
      | 78
      | 79
      | 80
      | 81
      | 82
      | 83
      | 84
      | 85
      | 86
      | 87
      | 88
      | 89
      | 90
      | 91
      | 92
      | 93
      | 94
      | 95
      | 96
      | 97
      | 98
      | 99
      | 100]
      Table=|
      | [7.50
      | 7.66
      | 7.80
      | 7.95
      | 8.10
      | 8.26
      | 8.43
      | 8.61
      | 8.80
      | 9.00
      | 9.20
      | 9.42
      | 9.64
      | 9.87
      | 10.11
      | 10.35
      | 10.60
      | 10.86
      | 11.12
      | 11.39
      | 11.67
      | 11.95
      | 12.24
      | 12.54
      | 12.84
      | 13.15
      | 13.46
      | 13.78
      | 14.10
      | 14.43
      | 14.77
      | 15.11
      | 15.45
      | 15.80
      | 16.16
      | 16.52
      | 16.88
      | 17.25
      | 17.63
      | 18.01
      | 18.39
      | 18.78
      | 19.17
      | 19.57
      | 19.98
      | 20.38
      | 20.79
      | 21.21
      | 21.63
      | 22.05
      | 22.48
      | 22.91
      | 23.35
      | 23.79
      | 24.23
      | 24.68
      | 25.14
      | 25.59
      | 26.05
      | 26.52
      | 26.98
      | 27.46
      | 27.93
      | 28.41
      | 28.89
      | 29.38
      | 29.87
      | 30.37
      | 30.86
      | 31.37
      | 31.87
      | 32.38
      | 32.89
      | 33.41
      | 33.92
      | 34.45
      | 34.97
      | 35.50
      | 36.03
      | 36.57
      | 37.11
      | 37.65
      | 38.20
      | 38.75
      | 39.30
      | 39.85
      | 40.41
      | 40.97
      | 41.54
      | 42.11
      | 42.68
      | 43.25
      | 43.83
      | 44.41
      | 45.00
      | 45.58
      | 46.17
      | 46.77
      | 47.36
      | 47.96]
  Constant : Constant  Value=0
  Gain : Gain  Gain=0.001
  Gain1 : Gain  Gain=0.001
  Logical Operator : Logic  Operator=OR  AllPortsSameDT=off
  Logical Operator1 : Logic  AllPortsSameDT=off
  Logical Operator2 : Logic  Operator=NOT  AllPortsSameDT=off
  Logical Operator3 : Logic  AllPortsSameDT=off
  Memory : Memory
  Relational Operator : RelationalOperator  Operator=<=  InputSameDT=off
  Relational Operator1 : RelationalOperator  InputSameDT=off
  Relational Operator2 : RelationalOperator  Operator=>  InputSameDT=off
  Rounding Function : Rounding
  Sterowanie zaworem : Outport
  wires:
  Nastawa/1 -> Rounding Function/1
  Char rusztu (set)/1 -> Gain/1  "%"
  Char rusztu (reset)/1 -> Gain1/1  "%"
  Relational Operator/1 -> Logical Operator/1
  Logical Operator/1 -> Memory/1, Logical Operator3/1
  Memory/1 -> Logical Operator1/1
  Logical Operator1/1 -> Logical Operator/2
  Relational Operator1/1 -> Logical Operator2/1
  Logical Operator2/1 -> Logical Operator1/2
  Pozycja rusztu/1 -> Relational Operator/1, Relational Operator1/1  "m"
  Logical Operator3/1 -> Sterowanie zaworem/1
  Relational Operator2/1 -> Logical Operator3/2
  Constant/1 -> Relational Operator2/2
  Gain/1 -> Relational Operator/2  "m"
  Gain1/1 -> Relational Operator1/2  "m"
  Rounding Function/1 -> Char rusztu (set)/1, Char rusztu (reset)/1, Relational Operator2/1

== system BrowarModel/System dozowania drozdzy/System dozowania drozdzy/Waga ==
  note: Waga
  note: Uszkodzenie mechanizmu
      | oprozniania wago
  Doplyw : Inport
  Oproznianie : Inport  Port=2
  Uszkodzenie oprozniania : Inport  Port=3
  1/Gestosc : Gain  Gain=1/1000
  Dot Product : DotProduct  OutDataTypeStr=Inherit: Inherit via internal rule
  Dynamika oprozniania : Gain  Gain=0.75
  Gestosc : Gain  Gain=1000
  Integrator : Integrator  LimitOutput=on  UpperSaturationLimit=100  LowerSaturationLimit=0
  Logical Operator : Logic  Operator=NOT  AllPortsSameDT=off
  Poz_dol : RelationalOperator  InputSameDT=off
  Poz_gora : RelationalOperator  Operator=<=  InputSameDT=off
  Pozycja dol : Constant  Value=0.9
  Pozycja gora : Constant  Value=0.1
  Product : Product  RndMeth=Zero
  Relay : Relay
  Relay1 : Relay
  Saturation : Saturate  UpperLimit=inf  LowerLimit=0
  Saturation1 : Saturate  UpperLimit=100  LowerLimit=0
  Sum : Sum  Inputs=|+-
  Sum1 : Sum
  Transfer Fcn : TransferFcn  Denominator=[1 1]
  Transport Delay : TransportDelay  DelayTime=1.5
  Wspolczynnik dynamiczny : Gain  Gain=.2
  Masa : Outport
  Odplyw chmielu : Outport  Port=2
  Poz dol : Outport  Port=3
  Poz gora : Outport  Port=4
  wires:
  Gestosc/1 -> Transport Delay/1  "kg/s"
  Transport Delay/1 -> Wspolczynnik dynamiczny/1, Sum/1
  Saturation/1 -> Gestosc/1  "m^3/s"
  Integrator/1 -> Dynamika oprozniania/1, Sum1/2
  Wspolczynnik dynamiczny/1 -> Sum1/1
  Doplyw/1 -> Saturation/1
  Sum1/1 -> Saturation1/1  "kg"
  Sum/1 -> Integrator/1
  Dot Product/1 -> Sum/2, 1/Gestosc/1
  Dynamika oprozniania/1 -> Dot Product/2
  1/Gestosc/1 -> Odplyw chmielu/1
  Saturation1/1 -> Masa/1  "kg"
  Poz_dol/1 -> Poz dol/1, Dot Product/1
  Poz_gora/1 -> Poz gora/1
  Pozycja dol/1 -> Poz_dol/2
  Pozycja gora/1 -> Poz_gora/2
  Transfer Fcn/1 -> Poz_dol/1, Poz_gora/1
  Oproznianie/1 -> Relay/1
  Uszkodzenie oprozniania/1 -> Relay1/1
  Relay1/1 -> Logical Operator/1
  Product/1 -> Transfer Fcn/1
  Relay/1 -> Product/1
  Logical Operator/1 -> Product/2

== system BrowarModel/System dozowania drozdzy/System dozowania drozdzy/Zasilacz hydrauliczny ==
  note: obr/min
  note: Zasilacz hydrauliczny
  note: Uszkodzenie:
      | Spadek cisnienia zasilania
  note: Uszkodzenie silnika pompy
  Zalaczenie pompy : Inport
  Przeplyw_pobor : Inport  Port=2
  Spadek cisnienia : Inport  Port=3
  Uszkodzenie silnika : Inport  Port=4
  Charakterystyka pompy F=f(P) (max 0.0001 m^3/s) : Lookup  InputValues=[0, 300]  Table=[0,0.0001]  SaturateOnIntegerOverflow=off
  Charakterystyka pompy P=f(obr) (max 300 kPa) : Lookup  InputValues=[0, 1440]  Table=[0,300]  SaturateOnIntegerOverflow=off
  Const1 : Constant  Value=100
  GUIMon : Gain
  Gain : Gain  Gain=1/100
  Gain1 : Gain  Gain=1/100
  Inercja wirnika : TransferFcn  Denominator=[0.5 1]
  Math Function : Math  Operator=square  SignedPower=on
  Obroty nominalne pompy : Gain  Gain=1440
  Opor : Gain  Gain=250 / ((0.0001)^2)
  Product1 : Product  RndMeth=Zero
  Relay : Relay  OnOutputValue=100
  Relay1 : Relay  OnOutputValue=0  OffOutputValue=1
  Sat uszk : Saturate  UpperLimit=100  LowerLimit=0
  Saturation : Saturate  UpperLimit=inf  LowerLimit=0
  Spadek obrotow pompy (od obciazenia) : Lookup  InputValues=[0, 300]  Table=[0,100]  SaturateOnIntegerOverflow=off
  Sum1 : Sum  Inputs=|+-
  Sum2 : Sum  Inputs=|+-
  Sum3 : Sum  Inputs=|+-
  Wplyw uszkodzenia : DotProduct  OutDataTypeStr=Inherit: Inherit via internal rule
  Max przeplyw zasilanie : Outport
  Cisnienie zasilania : Outport  Port=2
  wires:
  Obroty nominalne pompy/1 -> Sum2/1
  Sum2/1 -> Inercja wirnika/1
  Spadek obrotow pompy (od obciazenia)/1 -> Sum2/2  "obr/min"
  Inercja wirnika/1 -> Charakterystyka pompy P=f(obr) (max 300 kPa)/1  "obr/min"
  Charakterystyka pompy F=f(P) (max 0.0001 m^3/s)/1 -> Max przeplyw zasilanie/1  "m^3/s"
  Sum1/1 -> Saturation/1
  Opor/1 -> Sum1/2  "kPa"
  Saturation/1 -> Spadek obrotow pompy (od obciazenia)/1, Cisnienie zasilania/1, Charakterystyka pompy F=f(P) (max 0.0001 m^3/s)/1  "kPa"
  Math Function/1 -> Opor/1
  Zalaczenie pompy/1 -> Relay/1
  Przeplyw_pobor/1 -> Math Function/1
  Spadek cisnienia/1 -> Sat uszk/1
  Charakterystyka pompy P=f(obr) (max 300 kPa)/1 -> Product1/2  "kPa"
  Product1/1 -> Sum1/1  "kPa"
  Sat uszk/1 -> Sum3/2
  Const1/1 -> Sum3/1
  Sum3/1 -> Gain/1
  Wplyw uszkodzenia/1 -> Obroty nominalne pompy/1
  Relay/1 -> GUIMon/1
  Uszkodzenie silnika/1 -> Relay1/1
  Relay1/1 -> Wplyw uszkodzenia/2
  Gain/1 -> Product1/1
  GUIMon/1 -> Gain1/1
  Gain1/1 -> Wplyw uszkodzenia/1

== system BrowarModel/System dozowania drozdzy/System dozowania drozdzy/Zasobnik ==
  note: Zasobnik dozownika chmielu
  note: Uszkodzenie:
      | Wyciek z zasobnika dozownika
  Doplyw : Inport
  Odplyw : Inport  Port=2
  Wyciek : Inport  Port=3
  Char. zbiornika : Lookup  InputValues="[0.000\t0.003\t0.010\t0.023\t0.046\t0.079\t0.125\t0.186\t0.264\t0.362\t0.480\t0.622\t0.790\t0.972\t1.172\t1.372\t1.572\t1.772\t1.972\t2.172\t2.372\t2.572\t2.772\t2.972\t3.172\t3.372\t3.572\t3.772\t3.972\t4.172\t4.372\t4.572\t4.772\t4.972]"  Table="[0\t0.1\t0.2\t0.3\t0.4\t0.5\t0.6\t0.7\t0.8\t0.9\t1\t1.1\t1.2\t1.3\t1.4\t1.5\t1.6\t1.7\t1.8\t1.9\t2\t2.1\t2.2\t2.3\t2.4\t2.5\t2.6\t2.7\t2.8\t2.9\t3\t3.1\t3.2\t3.3]"  SaturateOnIntegerOverflow=off
  Detektory poziomu : Subsystem
  Integrator (max = 4.92m3) : Integrator  LimitOutput=on  UpperSaturationLimit=4.92  LowerSaturationLimit=0
  Max wyciek : Gain  Gain=0.01
  Product : Product  RndMeth=Zero
  Sat doplyw (F>=0) : Saturate  UpperLimit=inf  LowerLimit=0
  Sat odplyw (F>=0) : Saturate  UpperLimit=inf  LowerLimit=0
  Sat wyciek (0-1) : Saturate  UpperLimit=1  LowerLimit=0
  Sum : Sum  Inputs=|+-
  Sum1 : Sum  Inputs=|+-
  Wyciek char : Lookup  InputValues=[0, 0.5, 0.6, 1]  Table=[0, 0, 1, 1]  SaturateOnIntegerOverflow=off
  Poziom : Outport
  Poziom HI : Outport  Port=2
  Poziom LO : Outport  Port=3
  wires:
  Doplyw/1 -> Sat doplyw (F>=0)/1  "m3/s"
  Odplyw/1 -> Sat odplyw (F>=0)/1  "m3/s"
  Integrator (max = 4.92m3)/1 -> Char. zbiornika/1  "m3"
  Char. zbiornika/1 -> Poziom/1, Detektory poziomu/1(Poziom), Wyciek char/1  "m"
  Sat doplyw (F>=0)/1 -> Sum/1
  Sat odplyw (F>=0)/1 -> Sum/2
  Sum1/1 -> Integrator (max = 4.92m3)/1
  Sum/1 -> Sum1/1  "m3/s"
  Wyciek/1 -> Sat wyciek (0-1)/1  "[0,1]"
  Product/1 -> Sum1/2  "m3/h"
  Detektory poziomu/2(Poziom niski) -> Poziom LO/1
  Detektory poziomu/1(Poziom  wysoki) -> Poziom HI/1
  Sat wyciek (0-1)/1 -> Product/1
  Wyciek char/1 -> Max wyciek/1  "[0..1]"
  Max wyciek/1 -> Product/2  "m3/h"

== system BrowarModel/System dozowania drozdzy/System dozowania drozdzy/Zawor doplywu drozdzy ==
  note: Zawor doplywu slodu
  note: Uszkodzenie:
      | Brak materialu
  note: Uszkodzenie:
      | Dlawienie przeplywu w zaworze
  note: Uszkodzenie:
      | Przeciek wewnetrzny w zaworze
  note: Uszkodzenie:
      | Wyciek zewnetrzny w zaworze
  Sterowanie : Inport
  Dlawienie : Inport  Port=2
  Przeciek : Inport  Port=3
  Wyciek : Inport  Port=4
  Brak : Inport  Port=5
  Const : Constant  Value=100
  Const1 : Constant  Value=100
  Const2 : Constant  Value=100
  GUIMon : Gain
  Gain : Gain  Gain=1/100
  Gain1 : Gain  Gain=1/100
  Gain2 : Gain  Gain=1/100
  Integer Delay : Delay  DelayLength=15
  Napelnianie m3/s : Gain  Gain=Fmax/100
  Product : Product  RndMeth=Zero
  Product1 : Product  RndMeth=Zero
  Product2 : Product  RndMeth=Zero
  Relay : Relay  OnOutputValue=100
  Sat (0-100) : Saturate  UpperLimit=100  LowerLimit=0
  Sat dlawienie (0-100) : Saturate  UpperLimit=100  LowerLimit=0
  Sat przecieku (0-100) : Saturate  UpperLimit=100  LowerLimit=0
  Sat uszk (0-100) : Saturate  UpperLimit=100  LowerLimit=0
  Sat wyciek (0-100) : Saturate  UpperLimit=100  LowerLimit=0
  Sum : Sum  Inputs=|+-
  Sum1 : Sum  Inputs=|++
  Sum2 : Sum  Inputs=|+-
  Sum3 : Sum  Inputs=|+-
  Sum5 : Sum  Inputs=|++
  Transfer Fcn : TransferFcn  Denominator=[1 1]
  Zaklocenia : Subsystem
  Przeplyw : Outport
  wires:
  Product/1 -> Transfer Fcn/1  "m3/s"
  Const/1 -> Sum/1
  Sat dlawienie (0-100)/1 -> Sum/2
  Sum/1 -> Gain/1
  Transfer Fcn/1 -> Integer Delay/1  "m3/s"
  Sterowanie/1 -> Relay/1
  Dlawienie/1 -> Sat dlawienie (0-100)/1  "[0,100]"
  Sat (0-100)/1 -> Napelnianie m3/s/1
  Sum1/1 -> Sat (0-100)/1
  Relay/1 -> GUIMon/1
  Przeciek/1 -> Sat przecieku (0-100)/1
  Sat przecieku (0-100)/1 -> Sum1/2
  Wyciek/1 -> Sat wyciek (0-100)/1
  Const1/1 -> Sum2/1
  Sat wyciek (0-100)/1 -> Sum2/2
  Integer Delay/1 -> Product1/1  "m3/s"
  Product1/1 -> Przeplyw/1
  Sum2/1 -> Gain1/1
  Gain1/1 -> Product1/2
  Product2/1 -> Sum1/1
  GUIMon/1 -> Product2/2
  Brak/1 -> Sat uszk (0-100)/1
  Const2/1 -> Sum3/1
  Sat uszk (0-100)/1 -> Sum3/2
  Sum3/1 -> Gain2/1
  Napelnianie m3/s/1 -> Sum5/1, Zaklocenia/1(In)
  Sum5/1 -> Product/2
  Gain/1 -> Product/1
  Zaklocenia/1(Out) -> Sum5/2
  Gain2/1 -> Product2/1
